simulink model "modelling_completo_3D_LQR"  (R2020b)
settings: Solver=ode23tb  StartTime=0.0  StopTime=60  RelTol=1e-3
values from neighbouring files (symbols this model uses):
  U_star = [-m*g 0 0 0]    [Drone_Control_CASY_2.m]
  X_star = [0 0 0 0 10 0 0 0 0 0 0 0 0 0 0 0]    [Drone_Control_CASY_2.m]
undefined symbols (not defined in the file or in its folder): K_lqr
libraries: simulink x1
settings Model: SimulationMode=accelerator  Creator=edoardo  LastModifiedBy=edoardo
settings DebuggingCC: UnderSpecifiedDimensionMsg=warning

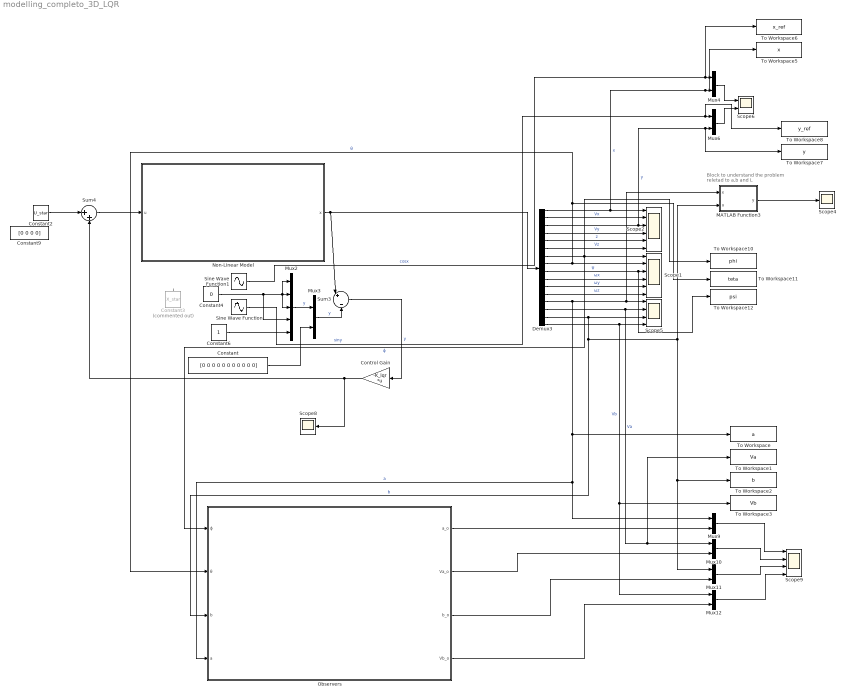
== system modelling_completo_3D_LQR ==
  note: Block to understand the problem reletad to a,b and L
  Constant : Constant  Value=[0 0 0 0 0 0 0 0 0 0 0]
  Constant2 : Constant  Value=U_star
  Constant3 : Constant  Commented=on  Value=X_star
  Constant4 : Constant  Value=0
  Constant6 : Constant
  Constant9 : Constant  Value=[0 0 0 0]
  Control Gain : Gain  Gain=-K_lqr  Multiplication=Matrix(K*u)
  Demux3 : Demux  Outputs=16
  MATLAB Function3 : MATLAB Function  TreatAsAtomicUnit=on
  Mux{3..4,6,9..12} (7 alike) : Mux  Inputs=2
  Mux2 : Mux  Inputs=5
  Non-Linear Model : Subsystem
  Observers : Subsystem
  Scope1 : Scope  NumInputPorts=6
  Scope2 : Scope  NumInputPorts=6
  Scope4 : Scope
  Scope5 : Scope  NumInputPorts=4
  Scope6 : Scope  NumInputPorts=2
  Scope8 : Scope
  Scope9 : Scope  NumInputPorts=4
  Sine Wave Function : Sin  Amplitude=0.5  Frequency=3  SampleTime=0
  Sine Wave Function1 : Sin  Amplitude=0.5  Frequency=3  Phase=pi/2  SampleTime=0
  Sum3 : Sum  Inputs=|+||-
  Sum4 : Sum  Inputs=|++
  To Workspace : ToWorkspace  VariableName=a  SampleTime=-1
  To Workspace1 : ToWorkspace  VariableName=Va  SampleTime=-1
  To Workspace10 : ToWorkspace  VariableName=phi  SampleTime=-1
  To Workspace11 : ToWorkspace  VariableName=teta  SampleTime=-1
  To Workspace12 : ToWorkspace  VariableName=psi  SampleTime=-1
  To Workspace2 : ToWorkspace  VariableName=b  SampleTime=-1
  To Workspace3 : ToWorkspace  VariableName=Vb  SampleTime=-1
  To Workspace5 : ToWorkspace  VariableName=x  SampleTime=-1
  To Workspace6 : ToWorkspace  VariableName=x_ref  SampleTime=-1
  To Workspace7 : ToWorkspace  VariableName=y  SampleTime=-1
  To Workspace8 : ToWorkspace  VariableName=y_ref  SampleTime=-1
  wires:
  Demux3/6 -> Scope2/6  "Vz"
  Demux3/5 -> Scope2/5  "z"
  Demux3/4 -> Scope2/4  "Vy"
  Demux3/2 -> Scope2/2  "Vx"
  Demux3/1 -> Scope2/1, To Workspace5/1, Mux4/2  "x"
  Demux3/3 -> To Workspace7/1, Mux6/2, Scope2/3  "y"
  Demux3/7 -> Observers/1(ϕ), Scope1/1, To Workspace10/1  "ϕ"
  Demux3/8 -> Observers/2(θ), To Workspace11/1, Scope1/2  "θ"
  Demux3/9 -> To Workspace12/1, Scope1/3  "ψ"
  Demux3/10 -> Scope1/4  "ωx"
  Demux3/11 -> Scope1/5  "ωy"
  Demux3/12 -> Scope1/6  "ωz"
  Demux3/13 -> Observers/4(a), Mux9/1, To Workspace/1, Scope5/1, MATLAB Function3/1(x)  "a"
  Demux3/14 -> Scope5/2, Mux10/1, To Workspace1/1  "Va"
  Demux3/15 -> Scope5/3, Observers/3(b), To Workspace2/1, Mux11/1, MATLAB Function3/2(u)  "b"
  Demux3/16 -> Scope5/4, Mux12/1, To Workspace3/1  "Vb"
  MATLAB Function3/1(y) -> Scope4/1
  Mux9/1 -> Scope9/1
  Mux10/1 -> Scope9/2
  Mux11/1 -> Scope9/3
  Mux12/1 -> Scope9/4
  Non-Linear Model/1(x) -> Sum3/1, Demux3/1
  Sum3/1 -> Control Gain/1  "y"
  Control Gain/1 -> Scope8/1, Sum4/2
  Sum4/1 -> Non-Linear Model/1(u)
  Constant3/1 -> ?
  Observers/1(a_o) -> Mux9/2
  Observers/2(Va_o) -> Mux10/2
  Observers/3(b_o) -> Mux11/2
  Observers/4(Vb_o) -> Mux12/2
  Constant4/1 -> Mux2/3, Mux2/2, Mux2/1, Mux2/4
  Mux2/1 -> Mux3/1  "y"
  Constant/1 -> Mux3/2
  Mux3/1 -> Sum3/2  "y"
  Sine Wave Function/1 -> To Workspace8/1, Mux6/1  "siny"
  Sine Wave Function1/1 -> To Workspace6/1, Mux4/1  "cosx"
  Mux4/1 -> Scope6/1
  Mux6/1 -> Scope6/2
  Constant6/1 -> Mux2/5
  Constant2/1 -> Sum4/1

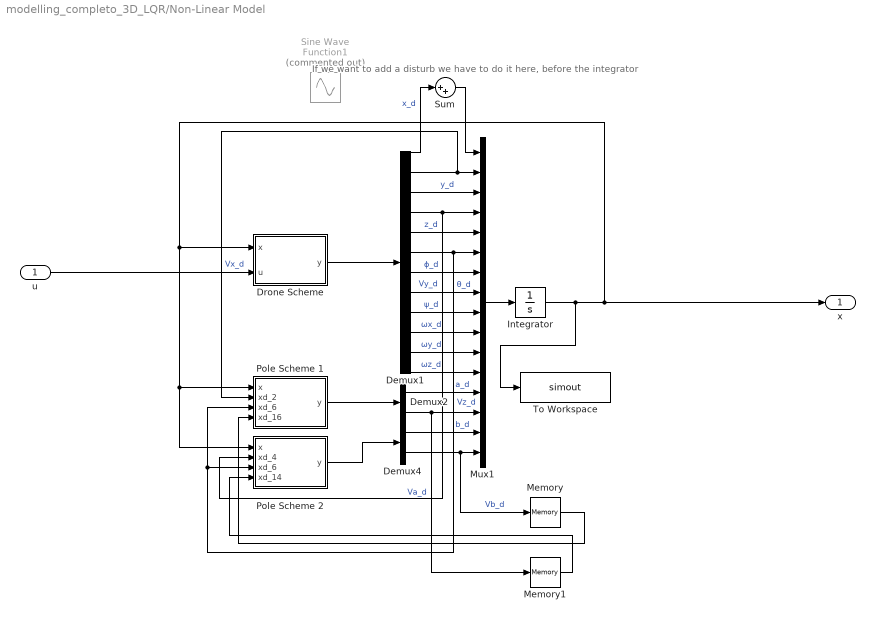
== system modelling_completo_3D_LQR/Non-Linear Model ==
  note: If we want to add a disturb we have to do it here, before the integrator
  u : Inport
  Demux1 : Demux  Outputs=12
  Demux2 : Demux  Outputs=2
  Demux4 : Demux  Outputs=2
  Drone Scheme : MATLAB Function  TreatAsAtomicUnit=on
  Integrator : Integrator  InitialCondition=[0 0 0 0 0 0 0 0 0 0 0 0 0 0 0 0]
  Memory : Memory
  Memory1 : Memory
  Mux1 : Mux  Inputs=16
  Pole Scheme 1 : MATLAB Function  TreatAsAtomicUnit=on
  Pole Scheme 2 : MATLAB Function  TreatAsAtomicUnit=on
  Sine Wave Function1 : Sin  Commented=on  Amplitude=0.5  Frequency=3  Phase=pi/2  SampleTime=0
  Sum : Sum  Inputs=|++
  To Workspace : ToWorkspace  VariableName=simout  SaveFormat=Timeseries  SampleTime=-1
  x : Outport
  wires:
  Demux1/9 -> Mux1/9  "ψ_d"
  Pole Scheme 1/1(y) -> Demux2/1
  Demux1/3 -> Mux1/3  "y_d"
  Memory1/1 -> Pole Scheme 2/4(xd_14)
  u/1 -> Drone Scheme/2(u)
  Demux4/2 -> Memory/1, Mux1/16  "Vb_d"
  Memory/1 -> Pole Scheme 1/4(xd_16)
  Demux2/2 -> Memory1/1, Mux1/14  "Va_d"
  Demux1/5 -> Mux1/5  "z_d"
  Mux1/1 -> Integrator/1
  Demux1/7 -> Mux1/7  "ϕ_d"
  Demux2/1 -> Mux1/13  "a_d"
  Demux1/11 -> Mux1/11  "ωy_d"
  Demux1/4 -> Pole Scheme 2/2(xd_4), Mux1/4  "Vy_d"
  Demux1/6 -> Pole Scheme 2/3(xd_6), Pole Scheme 1/3(xd_6), Mux1/6  "Vz_d"
  Integrator/1 -> x/1, Drone Scheme/1(x), Pole Scheme 2/1(x), Pole Scheme 1/1(x), To Workspace/1
  Demux1/1 -> Sum/1  "x_d"
  Demux4/1 -> Mux1/15  "b_d"
  Drone Scheme/1(y) -> Demux1/1
  Demux1/8 -> Mux1/8  "θ_d"
  Demux1/10 -> Mux1/10  "ωx_d"
  Pole Scheme 2/1(y) -> Demux4/1
  Demux1/2 -> Pole Scheme 1/2(xd_2), Mux1/2  "Vx_d"
  Demux1/12 -> Mux1/12  "ωz_d"
  Sum/1 -> Mux1/1

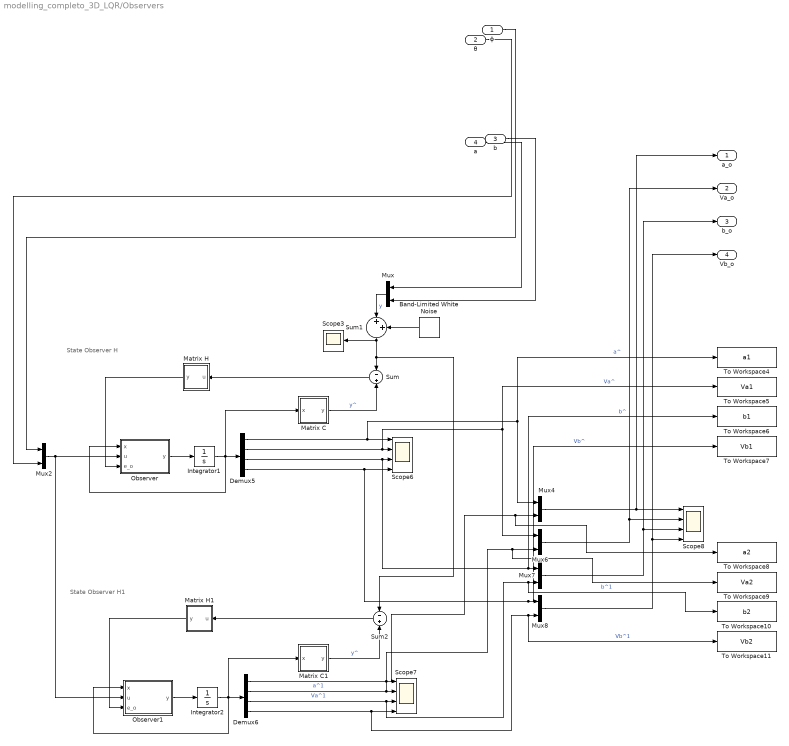
== system modelling_completo_3D_LQR/Observers ==
  note: State Observer H
  note: State Observer H1
  ϕ : Inport
  θ : Inport  Port=2
  b : Inport  Port=3
  a : Inport  Port=4
  Band-Limited White Noise : simulink/Sources/Band-Limited White Noise  Cov=[0.0001]  Ts=0.1  seed=[23341]
  Demux5 : Demux
  Demux6 : Demux
  Integrator1 : Integrator  InitialCondition=[0 0 0 0]
  Integrator2 : Integrator  InitialCondition=[0 0 0 0]
  Matrix C : MATLAB Function  TreatAsAtomicUnit=on
  Matrix C1 : MATLAB Function  TreatAsAtomicUnit=on
  Matrix H : MATLAB Function  TreatAsAtomicUnit=on
  Matrix H1 : MATLAB Function  TreatAsAtomicUnit=on
  Mux{,2,4,6..8} (6 alike) : Mux  Inputs=2
  Observer : MATLAB Function  TreatAsAtomicUnit=on
  Observer1 : MATLAB Function  TreatAsAtomicUnit=on
  Scope3 : Scope
  Scope6 : Scope  NumInputPorts=4
  Scope7 : Scope  NumInputPorts=4
  Scope8 : Scope  NumInputPorts=4
  Sum : Sum  Inputs=-+
  Sum1 : Sum  Inputs=|++
  Sum2 : Sum  Inputs=-+
  To Workspace10 : ToWorkspace  VariableName=b2  SampleTime=-1
  To Workspace11 : ToWorkspace  VariableName=Vb2  SampleTime=-1
  To Workspace4 : ToWorkspace  VariableName=a1  SampleTime=-1
  To Workspace5 : ToWorkspace  VariableName=Va1  SampleTime=-1
  To Workspace6 : ToWorkspace  VariableName=b1  SampleTime=-1
  To Workspace7 : ToWorkspace  VariableName=Vb1  SampleTime=-1
  To Workspace8 : ToWorkspace  VariableName=a2  SampleTime=-1
  To Workspace9 : ToWorkspace  VariableName=Va2  SampleTime=-1
  a_o : Outport
  Va_o : Outport  Port=2
  b_o : Outport  Port=3
  Vb_o : Outport  Port=4
  wires:
  ϕ/1 -> Mux2/1
  a/1 -> Mux/1
  Mux/1 -> Sum1/1  "y"
  Sum2/1 -> Matrix H1/1(u)
  Matrix H1/1(y) -> Observer1/3(e_o)
  θ/1 -> Mux2/2
  Sum1/1 -> Scope3/1, Sum2/1, Sum/1
  Mux8/1 -> Vb_o/1, Scope8/4
  Matrix H/1(y) -> Observer/3(e_o)
  Demux5/1 -> To Workspace4/1, Mux4/1, Scope6/1  "a^"
  Mux4/1 -> a_o/1, Scope8/1
  Mux7/1 -> b_o/1, Scope8/3
  Mux6/1 -> Va_o/1, Scope8/2
  Mux2/1 -> Observer/2(u), Observer1/2(u)
  Observer/1(y) -> Integrator1/1
  b/1 -> Mux/2
  Matrix C1/1(y) -> Sum2/2  "y^"
  Demux6/1 -> Mux4/2, To Workspace8/1, Scope7/1  "a^1"
  Integrator1/1 -> Demux5/1, Observer/1(x), Matrix C/1(x)
  Demux5/2 -> To Workspace5/1, Mux6/1, Scope6/2  "Va^"
  Demux6/4 -> Scope7/4, To Workspace11/1, Mux8/2  "Vb^1"
  Observer1/1(y) -> Integrator2/1
  Integrator2/1 -> Demux6/1, Matrix C1/1(x), Observer1/1(x)
  Demux6/2 -> Mux6/2, To Workspace9/1, Scope7/2  "Va^1"
  Demux5/4 -> Scope6/4, To Workspace7/1, Mux8/1  "Vb^"
  Matrix C/1(y) -> Sum/2  "y^"
  Demux5/3 -> To Workspace6/1, Mux7/1, Scope6/3  "b^"
  Sum/1 -> Matrix H/1(u)
  Demux6/3 -> To Workspace10/1, Mux7/2, Scope7/3  "b^1"
  Band-Limited White Noise/1 -> Sum1/2

== matlab function modelling_completo_3D_LQR/Non-Linear Model/Pole Scheme 1 ==
  data: x input; xd_2 input; y output; xd_6 input; xd_16 input
function y = fcn(x, xd_2,xd_6, xd_16) 
%Values of the parameters:
g=9.81; %acceleration of gravity in m/s^2
L=1; %Lenght of the pole in m

ZC=sqrt(L^2-(x(13))^2-(x(15))^2); %in the writehand notes is called with a greek letter
%Dynamics
xd_13=x(14);

xd_14=(1/(L^2-x(15)))*(-(x(13))^4*xd_2-(L^2-(x(15))^2)*xd_2-2*(x(13))^2*(x(15)*x(14)*x(16)+(-L^2+(x(15)^2))*xd_2)+(x(13))^3*((x(16))^2+x(15)*xd_16-ZC*(g+xd_6))+x(13)*(-L^2*x(15)*xd_16+(x(15))^3*xd_16+(x(15))^2*((x(14))^2-ZC*(g+xd_6))+L^2*(-(x(14))^2-(x(16))^2+ZC*(g+xd_6))));



y = [xd_13, xd_14];
% One output: y (12 components)

== matlab function modelling_completo_3D_LQR/Non-Linear Model/Drone Scheme ==
  data: x input; u input; y output
function y = fcn(x,u) %two inputs. One for the state variables the other one
%for the control inputs. I have 12 states and 4 inputs.

%Values of the parameters:

T=u(1);%Trust in Newton
m=1.55; %Mass in kg
tau_x=u(2);%Torque due to the airscrews 
tau_y=u(3);%Torque due to the airscrews 
tau_z=u(4);%Torque due to the airscrews

g=9.81; %acceleration of gravity in m/s^2
J_x=0.029145975;%inertia of the drone in kg*m^2
J_y=0.029418104;%inertia of the drone in kg*m^2
J_z=0.055519004;%inertia of the drone in kg*m^2


%Dynamics equations
xd_1=x(2);
xd_3=x(4);
xd_5=x(6);

xd_2=-(T/m)*(cos(x(7))*sin(x(8))*cos(x(9))+sin(x(7))*sin(x(9)));
xd_4=-(T/m)*(cos(x(7))*sin(x(8))*sin(x(9))-sin(x(7))*cos(x(9)));
xd_6=-g-(T/m)*(cos(x(7))*cos(x(8)));

xd_7=x(10)+tan(x(8))*(x(11)*sin(x(7))+x(12)*cos(x(7)));
xd_8=x(11)*cos(x(7))-x(12)*sin(x(7));
xd_9=x(11)*(sin(x(7))/cos(x(8)))+x(12)*(cos(x(7))/cos(x(8)));

xd_10=(tau_x+x(11)*x(12)*(J_z-J_y))/J_x;
xd_11=(tau_y+x(10)*x(12)*(J_x-J_z))/J_y;
xd_12=(tau_z+x(10)*x(11)*(J_y-J_x))/J_z;

%Rotation Matrix expressed thru the states x7,x8 and x9
%Rib = [cos(x(9))*cos(x(8)) cos(x(9))*sin(x(8))*sin(x(7))-sin(x(9))*cos(x(7)) cos(x(9))*sin(x(8))*cos(x(7))+sin(x(9))*sin(x(7));
%      sin(x(9))*cos(x(8)) sin(x(9))*sin(x(8))*sin(x(7))+cos(x(9))*cos(x(7)) sin(x(9))*sin(x(8))*cos(x(7))-cos(x(9))*sin(x(7));
%      -sin(x(8)) cos(x(8))*sin(x(7)) cos(x(8))*cos(x(7))];

y = [xd_1, xd_2, xd_3, xd_4, xd_5, xd_6, xd_7, xd_8, xd_9, xd_10, xd_11, xd_12];
% One output: y (12 components)

== matlab function modelling_completo_3D_LQR/Non-Linear Model/Pole Scheme 2 ==
  data: x input; xd_4 input; y output; xd_6 input; xd_14 input
function y = fcn(x, xd_4,xd_6, xd_14) 
%Values of the parameters:
g=9.81; %acceleration of gravity in m/s^2
L=1; %Lenght of the pole in m

ZC=sqrt(L^2-(x(13))^2-(x(15))^2); %in the writehand notes is called with a greek letter
%Dynamics
xd_15=x(16);

xd_16=(1/(L^2-x(13)))*(-(x(15))^4*xd_4-(L^2-(x(13))^2)*xd_4-2*(x(15))^2*(x(13)*x(14)*x(16)+(-L^2+(x(13)^2))*xd_4)+(x(15))^3*((x(14))^2+x(13)*xd_14-ZC*(g+xd_6))+x(15)*(-L^2*x(13)*xd_14+(x(13))^3*xd_14+(x(13))^2*((x(16))^2-ZC*(g+xd_6))+L^2*(-(x(14))^2-(x(16))^2+ZC*(g+xd_6))));



y = [xd_15, xd_16];
% One output: y (12 components)

== matlab function modelling_completo_3D_LQR/MATLAB Function3 ==
  data: x input; u input; y output
function y = fcn(x,u) 

y = 1^2-(x)^2-(u)^2;

== matlab function modelling_completo_3D_LQR/Observers/Observer ==
  data: x input; u input; y output; e_o input
function y = fcn(x,u,e_o)

g = 9.81;
L = 1;

Ap = [0 1 0 0;
      g/L 0 0 0;
      0 0 0 1;
      0 0 g/L 0];
%I will consider as inputs the dependence on x(7) and x(8), instead of the
%regular inputs that should be multiply for all zeros
Bp = [0 0;
      0 -g;
      0 0;
      g 0];
  
% Cp = [1 0 0 0;
%       0 0 1 0];
%  
% %I define the polynomial that contains the solutions I'd have as eigenvalues
% %of the matrix A+HC
% P = [-1 -5 -12 -2];
% 
% %https://it.mathworks.com/help/control/getstart/pole-placement.html
% H = -transpose(place(Ap',Cp',P));

  
% xd = transpose([0 0 0 0]);

xd = Ap*x+Bp*u+e_o;

y = xd;

== matlab function modelling_completo_3D_LQR/Observers/Matrix C ==
  data: x input; y output
function y = fcn(x)

Cp = [1 0 0 0;
      0 0 1 0];
y_o = Cp*x;

y = y_o;

== matlab function modelling_completo_3D_LQR/Observers/Matrix H ==
  data: u input; y output
function y = fcn(u)

H = [-7.6050 3.2173
    -18.7089 7.7697
    3.1895 -12.3950
    7.5755 -29.9089];

e_o = H*u;

y = e_o;

== matlab function modelling_completo_3D_LQR/Observers/Matrix H1 ==
  data: u input; y output
function y = fcn(u)

H1 = 1.0e+03*[-0.0603 0.0046;
              -0.5161 0.1104;
              0.0045 -0.1397;
              0.1083 -2.4035];
e_o = H1*u;

y = e_o;

== matlab function modelling_completo_3D_LQR/Observers/Observer1 ==
  data: x input; u input; y output; e_o input
function y = fcn(x,u,e_o)

g = 9.81;
L = 1;

Ap = [0 1 0 0;
      g/L 0 0 0;
      0 0 0 1;
      0 0 g/L 0];
   
   
Bp = [0 0;
      0 -g;
      0 0;
      g 0];
  
% Cp = [1 0 0 0;
%       0 0 1 0];
%  
% %I define the polynomial that contains the solutions I'd have as eigenvalues
% %of the matrix A+HC
% P = [-1 -5 -12 -2];
% 
% %https://it.mathworks.com/help/control/getstart/pole-placement.html
% H = -transpose(place(Ap',Cp',P));

  
% xd = transpose([0 0 0 0]);

xd = Ap*x+Bp*u+e_o;

y = xd;

== matlab function modelling_completo_3D_LQR/Observers/Matrix C1 ==
  data: x input; y output
function y = fcn(x)

Cp = [1 0 0 0;
      0 0 1 0];
y_o = Cp*x;

y = y_o;
